simulink model "Modele_LQR_6DOF"  (R2025b)
settings: Solver=VariableStepAuto  StartTime=0.0  StopTime=300  FixedStep=0.033333  RelTol=1e-3
values from neighbouring files (symbols this model uses):
  B = -234.459    [AUV_Params.sldd]    (also in block_compute_K.m = [ [                                          0,             )
  Fx1 = -14.142    [AUV_Params.sldd]
  Fx2 = -14.142    [AUV_Params.sldd]
  Fx3 = 0.0    [AUV_Params.sldd]
  Fx4 = 0.0    [AUV_Params.sldd]
  Fx5 = 0.0    [AUV_Params.sldd]
  Fx6 = 0.0    [AUV_Params.sldd]
  Fx7 = 14.142    [AUV_Params.sldd]
  Fx8 = 14.142    [AUV_Params.sldd]
  Fy1 = 14.142    [AUV_Params.sldd]
  Fy2 = -14.142    [AUV_Params.sldd]
  Fy3 = 0.0    [AUV_Params.sldd]
  Fy4 = 0.0    [AUV_Params.sldd]
  Fy5 = 0.0    [AUV_Params.sldd]
  Fy6 = 0.0    [AUV_Params.sldd]
  Fy7 = 14.142    [AUV_Params.sldd]
  Fy8 = -14.142    [AUV_Params.sldd]
  Fz1 = 0.0    [AUV_Params.sldd]
  Fz2 = 0.0    [AUV_Params.sldd]
  Fz3 = -20.0    [AUV_Params.sldd]
  Fz4 = -20.0    [AUV_Params.sldd]
  Fz5 = -20.0    [AUV_Params.sldd]
  Fz6 = -20.0    [AUV_Params.sldd]
  Fz7 = 0.0    [AUV_Params.sldd]
  Fz8 = 0.0    [AUV_Params.sldd]
  I_x = 0.578    [AUV_Params.sldd]
  I_y = 0.645    [AUV_Params.sldd]
  I_z = 0.9366    [AUV_Params.sldd]
  lx1 = 0.0194    [AUV_Params.sldd]
  lx2 = 0.0194    [AUV_Params.sldd]
  lx3 = -0.0317    [AUV_Params.sldd]
  lx4 = -0.0317    [AUV_Params.sldd]
  lx5 = 0.0317    [AUV_Params.sldd]
  lx6 = 0.0317    [AUV_Params.sldd]
  lx7 = -0.0194    [AUV_Params.sldd]
  lx8 = -0.0194    [AUV_Params.sldd]
  ly1 = 0.0381    [AUV_Params.sldd]
  ly2 = -0.0381    [AUV_Params.sldd]
  ly3 = 0.0049    [AUV_Params.sldd]
  ly4 = -0.0049    [AUV_Params.sldd]
  ly5 = 0.0049    [AUV_Params.sldd]
  ly6 = -0.0049    [AUV_Params.sldd]
  ly7 = 0.0381    [AUV_Params.sldd]
  ly8 = -0.0381    [AUV_Params.sldd]
  lz1 = 0.0575    [AUV_Params.sldd]
  lz2 = 0.0575    [AUV_Params.sldd]
  lz3 = 0.0366    [AUV_Params.sldd]
  lz4 = 0.0366    [AUV_Params.sldd]
  lz5 = 0.0366    [AUV_Params.sldd]
  lz6 = 0.0366    [AUV_Params.sldd]
  lz7 = 0.0575    [AUV_Params.sldd]
  lz8 = 0.0575    [AUV_Params.sldd]
  m = 23.9    [AUV_Params.sldd]
  W = 234.459    [AUV_Params.sldd]
  x_rb = 0.0    [AUV_Params.sldd]
  x_rg = 0.0    [AUV_Params.sldd]
  y_rb = 0.0    [AUV_Params.sldd]
  y_rg = 0.0    [AUV_Params.sldd]
  z_rb = 0.0    [AUV_Params.sldd]
  z_rg = 0.0    [AUV_Params.sldd]
undefined symbols (not defined in the file or in its folder): A_num, Q_envoyer, sigbuilder_block, SIZE_TRAJ, T_TRAJ, TRAJECTOIRE, YAW_MODE
libraries: simulink x12, sharedtransform x1, dspinverses x1, SignalEditorBlockLib x1
(part 1 of 4)
settings Model: DataDictionary=AUV_Params.sldd  Creator=ASUQTR  LastModifiedBy=louis
settings SolverCC: ZeroCrossAlgorithm=Adaptive  AlgebraicLoopSolver=TrustRegion
settings DebuggingCC: IgnoredZcDiagnostic=none  UnconnectedInputMsg=warning  UnconnectedOutputMsg=warning  UnconnectedLineMsg=warning
settings ModelReferenceCC: EnableRefExpFcnMdlSchedulingChecks=on
settings RTWCC: GPUComputeCapability=3.5  DLArmComputeVersion=19.05

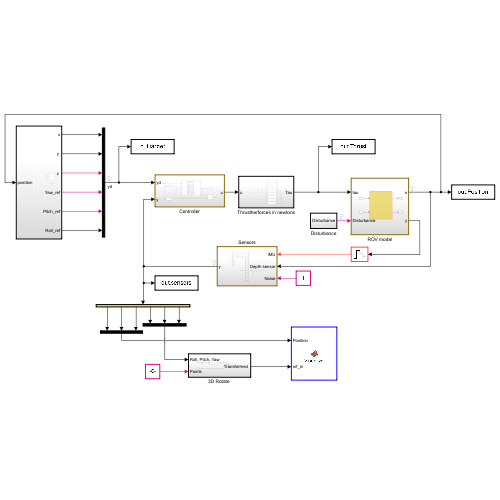
[thumbnail: Simulink's stored preview of the top-level diagram]
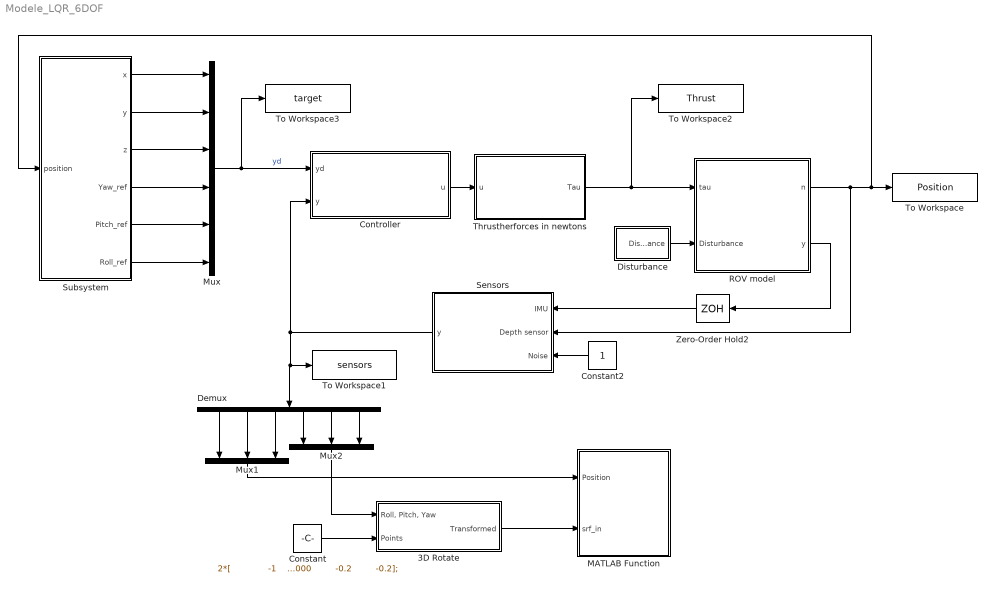
== system Modele_LQR_6DOF ==
  "3D Rotate " : Subsystem
  Constant : Constant  Value=|
      | 2*[              -1         -0.2         -0.2
      |     1.0000         -0.2         -0.2    
      | 1.0000    0.2000         -0.2
      |          -1    0.2000         -0.2
      |          -1         -0.2         -0.2
      |          -1         -0.2    0.2000
      |     1.0000         -0.2    0.2000
      |     1.0000    0.2000    0.2000
      |          -1    0.2000    0.2000
      |          -1         -0.2    0.2000
      |          -1   0.2000    0.2000
      |          -1    0.2000         -0.2
      |     1.0000    0.2000         -0.2
      |     1.0000    0.2000    0.2000
      |     1.0000         -0.2    0.2000
      |     1.0000         -0.2         -0.2];
  Constant2 : Constant
  Controller : Subsystem
  Demux : Demux  Outputs=6
  Disturbance : Subsystem
  MATLAB Function : MATLAB Function  TreatAsAtomicUnit=on  SystemSampleTime=0.05
  Mux : Mux  Inputs=6
  Mux1 : Mux  Inputs=3
  Mux2 : Mux  Inputs=3
  ROV model : Subsystem
  Sensors : Subsystem
  Subsystem : Subsystem
  Thrustherforces in newtons : Subsystem
  To Workspace : ToWorkspace  VariableName=Position  SaveFormat=Structure With Time  SampleTime=-1
  To Workspace1 : ToWorkspace  VariableName=sensors  SaveFormat=Structure With Time  SampleTime=-1
  To Workspace2 : ToWorkspace  VariableName=Thrust  SaveFormat=Structure With Time  SampleTime=-1
  To Workspace3 : ToWorkspace  VariableName=target  SaveFormat=Structure With Time  SampleTime=-1
  Zero-Order Hold2 : ZeroOrderHold  SampleTime=0.001
  wires:
  Mux/1 -> To Workspace3/1, Controller/1(yd)  "yd"
  Disturbance/1(Disturbance) -> ROV model/2(Disturbance)
  ROV model/1(n) -> Sensors/2(Depth sensor), Subsystem/1(position), To Workspace/1
  Thrustherforces in newtons/1(Tau) -> To Workspace2/1, ROV model/1(tau)
  Controller/1(u) -> Thrustherforces in newtons/1(u)
  Constant2/1 -> Sensors/3(Noise)
  Subsystem/2("y ") -> Mux/2
  Subsystem/1(x) -> Mux/1
  Subsystem/3("z ") -> Mux/3
  Subsystem/4(Yaw_ref) -> Mux/4
  Subsystem/5(Pitch_ref) -> Mux/5
  Subsystem/6(Roll_ref) -> Mux/6
  "3D Rotate "/1("Transformed ") -> MATLAB Function/2(srf_in)
  Constant/1 -> "3D Rotate "/2(Points)
  Demux/1 -> Mux1/1
  Demux/2 -> Mux1/2
  Demux/3 -> Mux1/3
  Mux1/1 -> MATLAB Function/1(Position)
  Demux/4 -> Mux2/1
  Demux/5 -> Mux2/2
  Demux/6 -> Mux2/3
  Mux2/1 -> "3D Rotate "/1("Roll, Pitch, Yaw")
  Sensors/1(y) -> To Workspace1/1, Demux/1, Controller/2(y)
  ROV model/2(y) -> Zero-Order Hold2/1
  Zero-Order Hold2/1 -> Sensors/1(IMU)

== system Modele_LQR_6DOF/3D Rotate  ==
  "Roll, Pitch, Yaw" : Inport
  Points : Inport  Port=2
  Gain : Gain
  Matrix Multiply : Product  Multiplication=Matrix(*)
  Rotation Angles to Direction Cosine Matrix : sharedtransform/Rotation Angles to Direction Cosine Matrix  rotationOrder=XYZ  aMode=aMode
  Transpose : Math  Operator=transpose  SignedPower=on
  "Transformed " : Outport  VectorParamsAs1DForOutWhenUnconnected=off
  wires:
  Matrix Multiply/1 -> "Transformed "/1
  Rotation Angles to Direction Cosine Matrix/1 -> Transpose/1
  Points/1 -> Matrix Multiply/1
  "Roll, Pitch, Yaw"/1 -> Gain/1
  Transpose/1 -> Matrix Multiply/2
  Gain/1 -> Rotation Angles to Direction Cosine Matrix/1

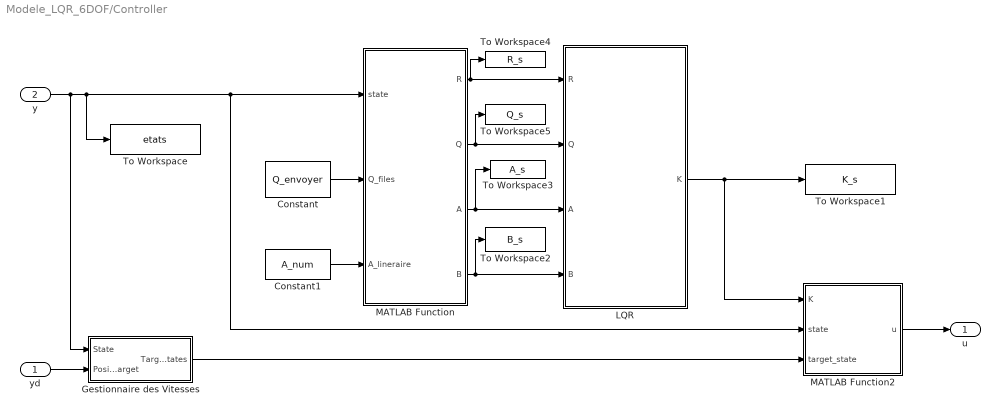
== system Modele_LQR_6DOF/Controller ==
  yd : Inport
  y : Inport  Port=2
  Constant : Constant  Value=Q_envoyer
  Constant1 : Constant  Value=A_num
  Gestionnaire des Vitesses : Subsystem
  LQR : Subsystem  Description=|  TreatAsAtomicUnit=on  mask(LQR with Algebric Riccati Equation){A=0, B=0, X0=0}
      | LQR Block
      | 
      | by Gurkan KAVURAN
      | gurkankavuran@gmail.com
      mask prompts: A "A (System Matrix)"; B "B (System Matrix)"; X0 "Xo (Initial Values of States)"
      mask help:
      | It is easy to optimize Q and R matrices with online process.
      | Please see the help file to define the block parameters.
      mask Help:
      | Parameters Example:
      | 
      | Q = diag([500 1 1 0 1 1] );
      | R = 1*diag([0.01 0.01 0.01 0.01]);
      | X0=[0 0 0 0 0 0;0 0 0 0 0 0;0 0 0 0 0 0;0 0 0 0 0 0;0 0 0 0 0 0;0 0 0 0 0 0];
      | 
      | "Matrix multiply" block is recommended to use in state feedback control mechanism.
      | 
      | 
      | http://www.gurkankavuran.com
      mask Display:
      | disp('LQR')
      | port_label('input', 1, 'R')
      | port_label('input', 2, 'Q')
      | port_label('input', 3, 'A')
      | port_label('input', 4, 'B')
      | port_label('output', 1, 'K')
  MATLAB Function : MATLAB Function  TreatAsAtomicUnit=on
  MATLAB Function2 : MATLAB Function  TreatAsAtomicUnit=on
  To Workspace : ToWorkspace  VariableName=etats  SaveFormat=Structure With Time  SampleTime=-1
  To Workspace1 : ToWorkspace  VariableName=K_s  SaveFormat=Structure With Time  SampleTime=-1
  To Workspace2 : ToWorkspace  VariableName=B_s  SaveFormat=Structure With Time  SampleTime=-1
  To Workspace3 : ToWorkspace  VariableName=A_s  SaveFormat=Structure With Time  SampleTime=-1
  To Workspace4 : ToWorkspace  VariableName=R_s  SaveFormat=Structure With Time  SampleTime=-1
  To Workspace5 : ToWorkspace  VariableName=Q_s  SaveFormat=Structure With Time  SampleTime=-1
  u : Outport
  wires:
  MATLAB Function/4(B) -> LQR/4(B), To Workspace2/1
  MATLAB Function/2(Q) -> LQR/2(Q), To Workspace5/1
  LQR/1(K) -> MATLAB Function2/1(K), To Workspace1/1
  y/1 -> Gestionnaire des Vitesses/1(State), To Workspace/1, MATLAB Function2/2(state), MATLAB Function/1(state)
  MATLAB Function/1(R) -> LQR/1(R), To Workspace4/1
  yd/1 -> Gestionnaire des Vitesses/2(Position_target)
  Gestionnaire des Vitesses/1(Target_states) -> MATLAB Function2/3(target_state)
  MATLAB Function/3(A) -> LQR/3(A), To Workspace3/1
  Constant/1 -> MATLAB Function/2(Q_files)
  Constant1/1 -> MATLAB Function/3(A_lineraire)
  MATLAB Function2/1(u) -> u/1

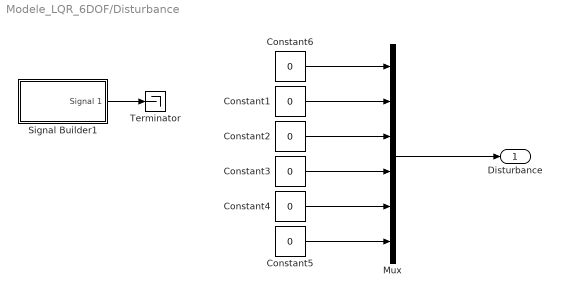
== system Modele_LQR_6DOF/Disturbance ==
  Constant{1..6} (6 alike) : Constant  Value=0
  Mux : Mux  Inputs=6
  Signal Builder1 : Subsystem  Tag=STV Subsys  LoadFcn=sigbuilder_block('load');  StartFcn=sigbuilder_block('start');  StopFcn=sigbuilder_block('stop');  ClipboardFcn=sigbuilder_block('clipboard');  mask(Sigbuilder block){tuvar=[0:10]}
      mask help: Simulink:masks:SigbuilderBlock_MD
      mask init:
      | if ~strcmp(get_param(bdroot(gcbh),'SimulationStatus'),'stopped') tuvar = sigbuilder_block('maskInit'); end
      settings: CopyFcn=sigbuilder_block('copy');  DeleteFcn=sigbuilder_block('delete');  ModelCloseFcn=sigbuilder_block('modelClose');  PreSaveFcn=sigbuilder_block('preSave');  PauseFcn=sigbuilder_block('pause');  ContinueFcn=sigbuilder_block('continue');  NameChangeFcn=sigbuilder_block('namechange');  OpenFcn=sigbuilder_block('open',[252.75 107.25 644.25 387.75 ]);  CloseFcn=sigbuilder_block('close');
      mask Display: plot(0, 0, 100, 100,[2, 2, 32, 32, 2], [68, 8, 8, 68, 68],[32, 2], [38, 38], [32, 19, 2],[53, 60, 44], [32, 17, 17, 2],[16, 16, 31, 31]);txt = getActiveGroup(gcbh);text(2, 100, txt,'verticalAlignment', 'top');
  Terminator : Terminator
  Disturbance : Outport
  wires:
  Mux/1 -> Disturbance/1
  Constant1/1 -> Mux/2
  Constant2/1 -> Mux/3
  Constant4/1 -> Mux/5
  Constant5/1 -> Mux/6
  Constant3/1 -> Mux/4
  Constant6/1 -> Mux/1
  Signal Builder1/1(Signal 1) -> Terminator/1

== system Modele_LQR_6DOF/ROV model ==
  tau : Inport
  Disturbance : Inport  Port=2
  ROV model : Subsystem
  n : Outport
  y : Outport  Port=2
  wires:
  tau/1 -> ROV model/1(tau)
  Disturbance/1 -> ROV model/2(Disturbance)
  ROV model/2(euler+vitesse_body) -> y/1
  ROV model/1(𝜂) -> n/1

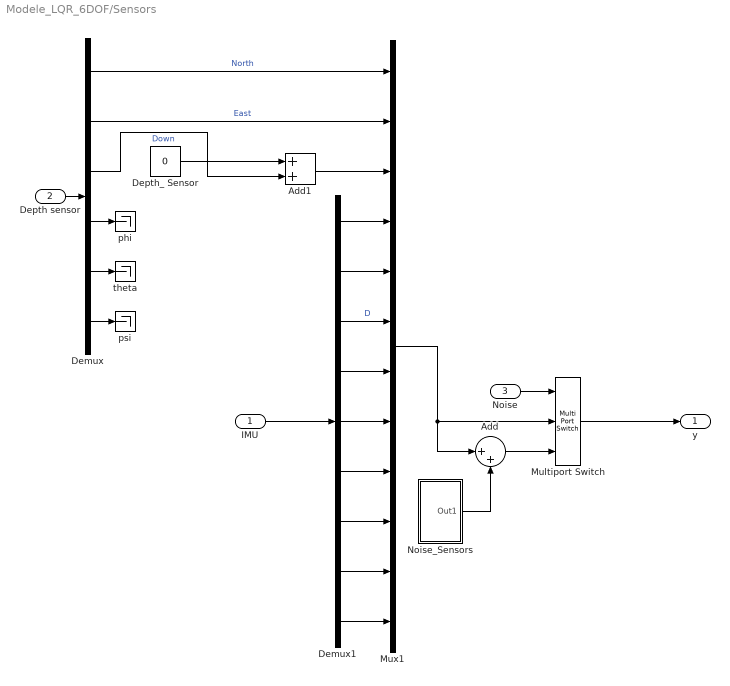
== system Modele_LQR_6DOF/Sensors ==
  IMU : Inport
  Depth sensor : Inport  Port=2
  Noise : Inport  Port=3
  Add : Sum  Inputs=|++
  Add1 : Sum
  Demux : Demux  Outputs=6
  Demux1 : Demux  Outputs=9
  Depth_ Sensor : Constant  Value=0
  Multiport Switch : MultiPortSwitch  Inputs=2  SaturateOnIntegerOverflow=off  InputSameDT=off
  Mux1 : Mux  Inputs=12
  Noise_Sensors : Subsystem
  phi : Terminator
  psi : Terminator
  theta : Terminator
  y : Outport
  wires:
  Multiport Switch/1 -> y/1
  Add/1 -> Multiport Switch/3
  Noise/1 -> Multiport Switch/1
  Mux1/1 -> Multiport Switch/2, Add/1
  Depth sensor/1 -> Demux/1
  Demux/4 -> phi/1
  Demux/5 -> theta/1
  Demux/6 -> psi/1
  Demux/3 -> Add1/2  "Down"
  Depth_ Sensor/1 -> Add1/1
  IMU/1 -> Demux1/1
  Add1/1 -> Mux1/3
  Demux/2 -> Mux1/2  "East"
  Demux/1 -> Mux1/1  "North"
  Demux1/1 -> Mux1/4
  Demux1/2 -> Mux1/5
  Demux1/3 -> Mux1/6  "D"
  Demux1/4 -> Mux1/7
  Demux1/5 -> Mux1/8
  Demux1/6 -> Mux1/9
  Demux1/7 -> Mux1/10
  Demux1/8 -> Mux1/11
  Demux1/9 -> Mux1/12
  Noise_Sensors/1(Out1) -> Add/2

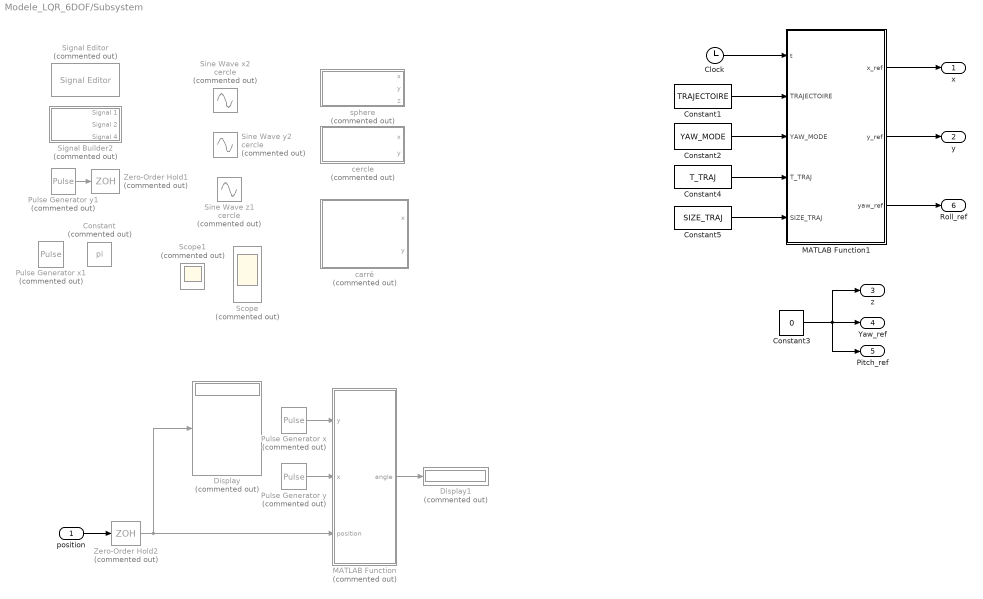
== system Modele_LQR_6DOF/Subsystem ==
  position : Inport
  Clock : Clock
  Constant : Constant  Commented=on  Value=pi
  Constant1 : Constant  Value=TRAJECTOIRE
  Constant2 : Constant  Value=YAW_MODE
  Constant3 : Constant  Value=0
  Constant4 : Constant  Value=T_TRAJ
  Constant5 : Constant  Value=SIZE_TRAJ
  Display : Display  Commented=on
  Display1 : Display  Commented=on
  MATLAB Function : MATLAB Function  Commented=on  TreatAsAtomicUnit=on
  MATLAB Function1 : MATLAB Function  TreatAsAtomicUnit=on
  Pulse Generator x : DiscretePulseGenerator  Commented=on  PulseType=Time based  Amplitude=2  Period=30  PulseWidth=50
  Pulse Generator x1 : DiscretePulseGenerator  Commented=on  PulseType=Time based  Amplitude=pi  Period=30  PulseWidth=50
  Pulse Generator y : DiscretePulseGenerator  Commented=on  PulseType=Time based  Amplitude=2  Period=30  PulseWidth=50  PhaseDelay=7.5
  Pulse Generator y1 : DiscretePulseGenerator  Commented=on  PulseType=Time based  Amplitude=pi/2  Period=30  PulseWidth=50  PhaseDelay=7.5
  Scope : Scope  Commented=on  NumInputPorts=3
      settings: ActiveDisplayYMinimum=-0.25  ActiveDisplayYMaximum=2.25
  Scope1 : Scope  Commented=on  NumInputPorts=2
      settings: ActiveDisplayYMinimum=-1  ActiveDisplayYMaximum=1
  Signal Builder2 : Subsystem  Tag=STV Subsys  Commented=on  LoadFcn=sigbuilder_block('load');  StartFcn=sigbuilder_block('start');  StopFcn=sigbuilder_block('stop');  ClipboardFcn=sigbuilder_block('clipboard');  mask(Sigbuilder block){tuvar=[0:10]}
      mask help: Simulink:masks:SigbuilderBlock_MD
      mask init:
      | if ~strcmp(get_param(bdroot(gcbh),'SimulationStatus'),'stopped') tuvar = sigbuilder_block('maskInit'); end
      settings: CopyFcn=sigbuilder_block('copy');  DeleteFcn=sigbuilder_block('delete');  ModelCloseFcn=sigbuilder_block('modelClose');  PreSaveFcn=sigbuilder_block('preSave');  PauseFcn=sigbuilder_block('pause');  ContinueFcn=sigbuilder_block('continue');  NameChangeFcn=sigbuilder_block('namechange');  OpenFcn=sigbuilder_block('open',[566.25 108.75 550.5 372.75 ]);  CloseFcn=sigbuilder_block('close');
      mask Display: plot(0, 0, 100, 100,[2, 2, 32, 32, 2], [68, 8, 8, 68, 68],[32, 2], [38, 38], [32, 19, 2],[53, 60, 44], [32, 17, 17, 2],[16, 16, 31, 31]);txt = getActiveGroup(gcbh);text(2, 100, txt,'verticalAlignment', 'top');
  Signal Editor : SignalEditorBlockLib/Signal Editor  Commented=on  FileName=sous marin en pentagone.mat  ActiveScenario=Scenario  ActiveSignal=Signal X  IsBus=off  OutputBusObjectStr=Bus: BusObject  SampleTime=0  Interpolate=off  ZeroCross=off  OutputAfterFinalValue=Setting to zero  Unit=inherit  PreserveSignalName=on  ApplySigPropsToAllScenarios=on  ApplySigPropsToAllSignals=off  SignalPropertySource=Dialog parameters
  Sine Wave x2 cercle : Sin  Commented=on  Amplitude=2  Frequency=0.48541  Phase=pi/2  SampleTime=0
  Sine Wave y2 cercle : Sin  Commented=on  Amplitude=2  Frequency=0.48541  SampleTime=0
  Sine Wave z1 cercle : Sin  Commented=on  Amplitude=2  Frequency=0.3  Phase=pi/2  SampleTime=0
  Zero-Order Hold1 : ZeroOrderHold  Commented=on  SampleTime=8
  Zero-Order Hold2 : ZeroOrderHold  Commented=on
  carré : Subsystem  Commented=on
  cercle : Subsystem  Commented=on
  sphere : Subsystem  Commented=on
  x : Outport  VectorParamsAs1DForOutWhenUnconnected=off
  "y " : Outport  Port=2  VectorParamsAs1DForOutWhenUnconnected=off
  "z " : Outport  Port=3  VectorParamsAs1DForOutWhenUnconnected=off
  Yaw_ref : Outport  Port=4  VectorParamsAs1DForOutWhenUnconnected=off
  Pitch_ref : Outport  Port=5  VectorParamsAs1DForOutWhenUnconnected=off
  Roll_ref : Outport  Port=6  VectorParamsAs1DForOutWhenUnconnected=off
  wires:
  Pulse Generator x/1 -> MATLAB Function/1(y)
  position/1 -> Zero-Order Hold2/1
  Zero-Order Hold2/1 -> Display/1, MATLAB Function/3(position)
  MATLAB Function/1(angle) -> Display1/1
  Pulse Generator y/1 -> MATLAB Function/2(x)
  Pulse Generator y1/1 -> Zero-Order Hold1/1
  Constant3/1 -> Yaw_ref/1, "z "/1, Pitch_ref/1
  Clock/1 -> MATLAB Function1/1(t)
  MATLAB Function1/1(x_ref) -> x/1
  MATLAB Function1/2(y_ref) -> "y "/1
  Constant1/1 -> MATLAB Function1/2(TRAJECTOIRE)
  Constant2/1 -> MATLAB Function1/3(YAW_MODE)
  MATLAB Function1/3(yaw_ref) -> Roll_ref/1
  Constant4/1 -> MATLAB Function1/4(T_TRAJ)
  Constant5/1 -> MATLAB Function1/5(SIZE_TRAJ)

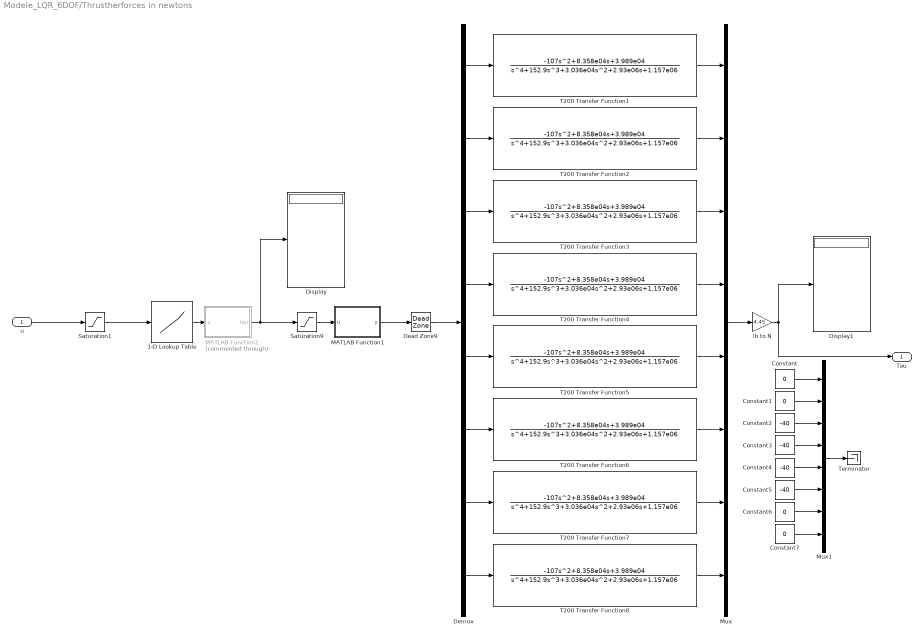
== system Modele_LQR_6DOF/Thrustherforces in newtons ==
  u : Inport
  1-D Lookup Table : Lookup_n-D  NumberOfTableDimensions=1  BreakpointsForDimension1=[-1:0.01:1]  Table=1500 + 400 * ([-1:0.01:1])  InternalRulePriority=Speed  RndMeth=Simplest
  Constant{,1,6..7} (4 alike) : Constant  Value=0
  Constant{2..5} (4 alike) : Constant  Value=-40
  Dead Zone9 : DeadZone  LowerValue=-10  UpperValue=+10
  Demux : Demux  Outputs=8
  Display : Display
  Display1 : Display
  MATLAB Function1 : MATLAB Function  TreatAsAtomicUnit=on
  MATLAB Function2 : MATLAB Function  Commented=through  TreatAsAtomicUnit=on
  Mux : Mux  Inputs=8
  Mux1 : Mux  Inputs=8
  Saturation1 : Saturate  UpperLimit=1  LowerLimit=-1
  Saturation9 : Saturate  UpperLimit=1900  LowerLimit=1100
  T200 Transfer Function{1..8} (8 alike) : TransferFcn  Numerator="[-107  8.358e04  3.989e04]"  Denominator="[1 152.9  3.036e04  2.93e06  1.157e06]"
  Terminator : Terminator
  lb to N : Gain  Gain=4.45
  Tau : Outport
  wires:
  u/1 -> Saturation1/1
  1-D Lookup Table/1 -> MATLAB Function2/1(u)
  Dead Zone9/1 -> Demux/1
  T200 Transfer Function1/1 -> Mux/1
  T200 Transfer Function5/1 -> Mux/5
  T200 Transfer Function7/1 -> Mux/7
  T200 Transfer Function8/1 -> Mux/8
  Mux/1 -> lb to N/1
  lb to N/1 -> Display1/1, Tau/1
  Saturation9/1 -> MATLAB Function1/1(u)
  MATLAB Function1/1(y) -> Dead Zone9/1
  MATLAB Function2/1(tau) -> Display/1, Saturation9/1
  Constant/1 -> Mux1/1
  Constant1/1 -> Mux1/2
  Constant2/1 -> Mux1/3
  Constant3/1 -> Mux1/4
  Constant4/1 -> Mux1/5
  Constant5/1 -> Mux1/6
  Constant6/1 -> Mux1/7
  Constant7/1 -> Mux1/8
  Demux/1 -> T200 Transfer Function1/1
  Demux/2 -> T200 Transfer Function2/1
  Demux/3 -> T200 Transfer Function3/1
  Demux/4 -> T200 Transfer Function4/1
  Demux/5 -> T200 Transfer Function5/1
  Demux/6 -> T200 Transfer Function6/1
  Demux/7 -> T200 Transfer Function7/1
  Demux/8 -> T200 Transfer Function8/1
  T200 Transfer Function6/1 -> Mux/6
  T200 Transfer Function2/1 -> Mux/2
  T200 Transfer Function3/1 -> Mux/3
  T200 Transfer Function4/1 -> Mux/4
  Saturation1/1 -> 1-D Lookup Table/1
  Mux1/1 -> Terminator/1

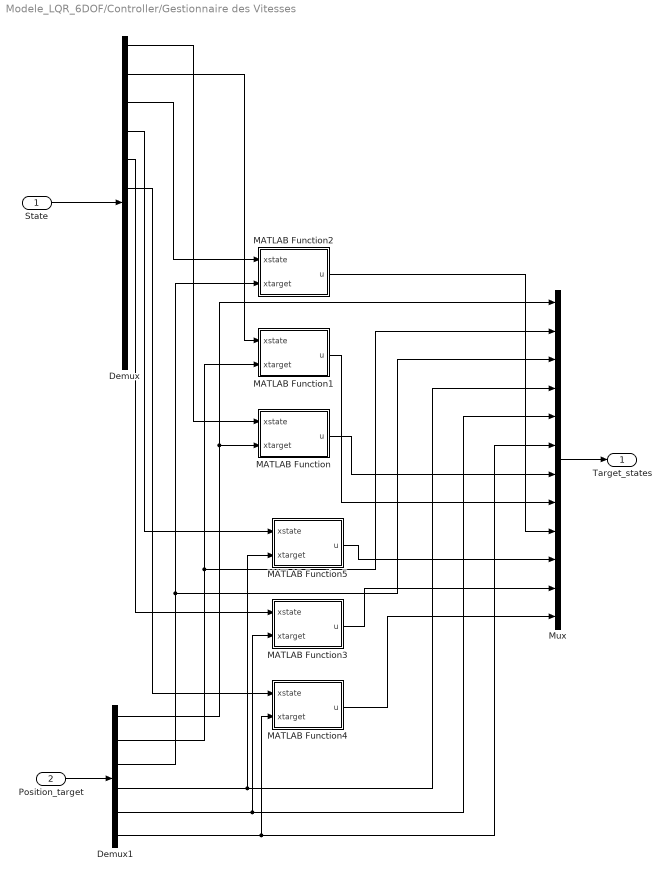
== system Modele_LQR_6DOF/Controller/Gestionnaire des Vitesses ==
  State : Inport
  Position_target : Inport  Port=2
  Demux : Demux  Outputs=12
  Demux1 : Demux  Outputs=6
  MATLAB Function : MATLAB Function  TreatAsAtomicUnit=on
  MATLAB Function1 : MATLAB Function  TreatAsAtomicUnit=on
  MATLAB Function2 : MATLAB Function  TreatAsAtomicUnit=on
  MATLAB Function3 : MATLAB Function  TreatAsAtomicUnit=on
  MATLAB Function4 : MATLAB Function  TreatAsAtomicUnit=on
  MATLAB Function5 : MATLAB Function  TreatAsAtomicUnit=on
  Mux : Mux  Inputs=12
  Target_states : Outport
  wires:
  State/1 -> Demux/1
  Position_target/1 -> Demux1/1
  Mux/1 -> Target_states/1
  Demux1/4 -> MATLAB Function5/2(xtarget), Mux/4
  Demux1/5 -> MATLAB Function3/2(xtarget), Mux/5
  Demux1/6 -> MATLAB Function4/2(xtarget), Mux/6
  Demux1/2 -> MATLAB Function1/2(xtarget), Mux/2
  Demux1/3 -> MATLAB Function2/2(xtarget), Mux/3
  MATLAB Function2/1(u) -> Mux/9
  MATLAB Function1/1(u) -> Mux/8
  Demux/1 -> MATLAB Function/1(xstate)
  Demux1/1 -> Mux/1, MATLAB Function/2(xtarget)
  MATLAB Function/1(u) -> Mux/7
  Demux/2 -> MATLAB Function1/1(xstate)
  Demux/3 -> MATLAB Function2/1(xstate)
  Demux/4 -> MATLAB Function5/1(xstate)
  Demux/5 -> MATLAB Function3/1(xstate)
  Demux/6 -> MATLAB Function4/1(xstate)
  MATLAB Function4/1(u) -> Mux/12
  MATLAB Function3/1(u) -> Mux/11
  MATLAB Function5/1(u) -> Mux/10

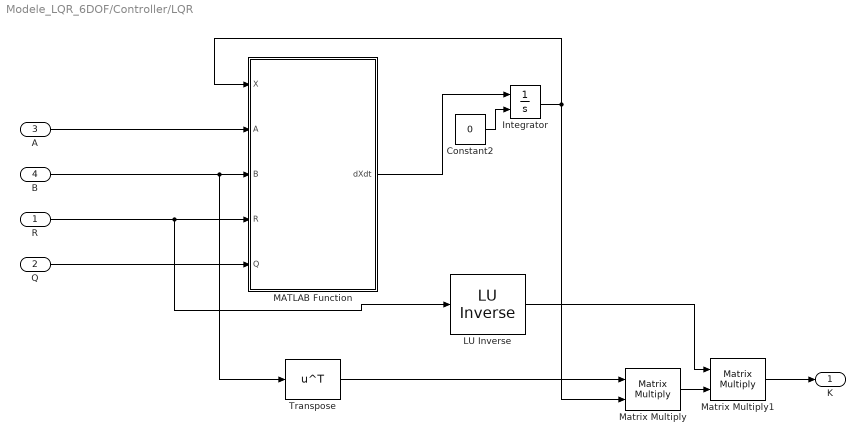
== system Modele_LQR_6DOF/Controller/LQR ==
  R : Inport
  Q : Inport  Port=2
  A : Inport  Port=3
  B : Inport  Port=4
  " LU Inverse" : dspinverses/ LU Inverse
  Constant2 : Constant  Value=0
  Integrator : Integrator  InitialConditionSource=external  InitialCondition=[1 1 1 1 1 1 1 1 1 1 1 1 1 1 1 1 1 1 1 1 1 1 1 1 1 1 1 1 1 1 1 1 1 1 1 1]
  MATLAB Function : MATLAB Function  TreatAsAtomicUnit=on
  Matrix Multiply : Product  Multiplication=Matrix(*)
  Matrix Multiply1 : Product  Multiplication=Matrix(*)
  Transpose : Math  Operator=transpose
  K : Outport
  wires:
  Matrix Multiply1/1 -> K/1
  A/1 -> MATLAB Function/2(A)
  B/1 -> Transpose/1, MATLAB Function/3(B)
  " LU Inverse"/1 -> Matrix Multiply1/1
  Constant2/1 -> Integrator/2
  Matrix Multiply/1 -> Matrix Multiply1/2
  Transpose/1 -> Matrix Multiply/1
  Integrator/1 -> Matrix Multiply/2, MATLAB Function/1(X)
  Q/1 -> MATLAB Function/5(Q)
  R/1 -> " LU Inverse"/1, MATLAB Function/4(R)
  MATLAB Function/1(dXdt) -> Integrator/1

== system Modele_LQR_6DOF/Disturbance/Signal Builder1 ==
  Demux : Demux  Tag=STV Demux  Outputs=1
      settings: DisplayOption=none
  FromWs : FromWorkspace  Tag=STV FromWs  VariableName=tuvar
      SigBuilderData=|
      | common.afterFinalStr = 'Extrapolate'
      | common.sampleTime = 0
      | dataSet.timeRange = [0 20]
      | dataSet.name = 'Group 1'
      | sbobj.Groups.Name = 'Group 1'
      | sbobj.Groups.Signals.Name = 'Signal 1'
      | sbobj.Groups.Signals.XData = [0 2 20]
      | sbobj.Groups.Signals.YData = [0 1 1]
      | sbobj.Groups.TimeRange = [0 20]
  Signal 1 : Outport  Tag=STV Outport
  wires:
  FromWs/1 -> Demux/1
  Demux/1 -> Signal 1/1

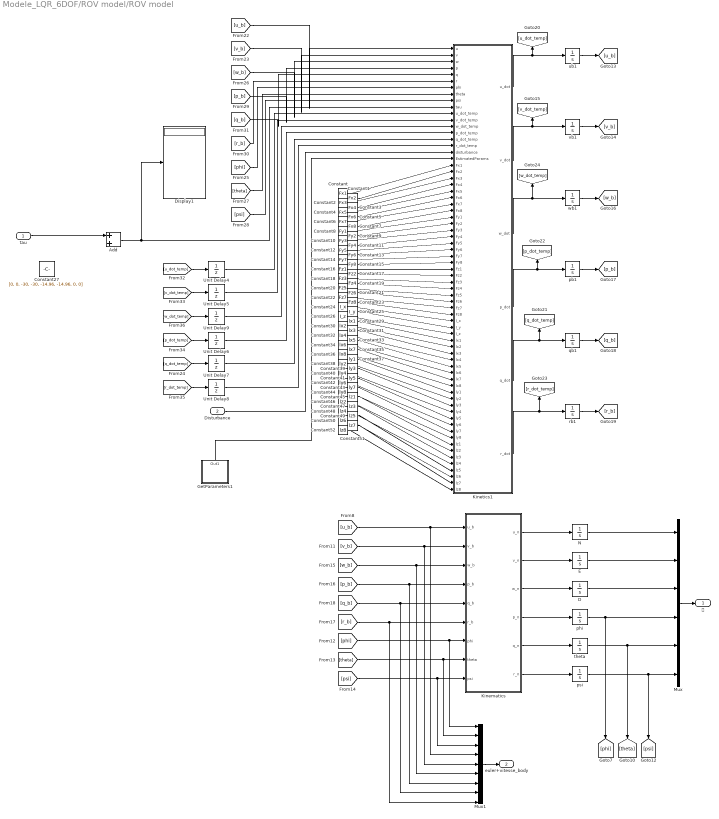
== system Modele_LQR_6DOF/ROV model/ROV model ==
  tau : Inport
  Disturbance : Inport  Port=2
  Add : Sum
  Constant : Constant  Value=Fx1
  Constant1 : Constant  Value=Fx2
  Constant10 : Constant  Value=Fy3
  Constant11 : Constant  Value=Fy4
  Constant12 : Constant  Value=Fy5
  Constant13 : Constant  Value=Fy6
  Constant14 : Constant  Value=Fy7
  Constant15 : Constant  Value=Fy8
  Constant16 : Constant  Value=Fz1
  Constant17 : Constant  Value=Fz2
  Constant18 : Constant  Value=Fz3
  Constant19 : Constant  Value=Fz4
  Constant2 : Constant  Value=Fx3
  Constant20 : Constant  Value=Fz5
  Constant21 : Constant  Value=Fz6
  Constant22 : Constant  Value=Fz7
  Constant23 : Constant  Value=Fz8
  Constant24 : Constant  Value=I_x
  Constant25 : Constant  Value=I_y
  Constant26 : Constant  Value=I_z
  Constant27 : Constant  Value=[0, 0, -30, -30, -14.96, -14.96, 0, 0]
  Constant29 : Constant  Value=lx1
  Constant3 : Constant  Value=Fx4
  Constant30 : Constant  Value=lx2
  Constant31 : Constant  Value=lx3
  Constant32 : Constant  Value=lx4
  Constant33 : Constant  Value=lx5
  Constant34 : Constant  Value=lx6
  Constant35 : Constant  Value=lx7
  Constant36 : Constant  Value=lx8
  Constant37 : Constant  Value=ly1
  Constant38 : Constant  Value=ly2
  Constant39 : Constant  Value=ly3
  Constant4 : Constant  Value=Fx5
  Constant40 : Constant  Value=ly4
  Constant41 : Constant  Value=ly5
  Constant42 : Constant  Value=ly6
  Constant43 : Constant  Value=ly7
  Constant44 : Constant  Value=ly8
  Constant45 : Constant  Value=lz1
  Constant46 : Constant  Value=lz2
  Constant47 : Constant  Value=lz3
  Constant48 : Constant  Value=lz4
  Constant49 : Constant  Value=lz5
  Constant5 : Constant  Value=Fx6
  Constant50 : Constant  Value=lz6
  Constant51 : Constant  Value=lz7
  Constant52 : Constant  Value=lz8
  Constant6 : Constant  Value=Fx7
  Constant7 : Constant  Value=Fx8
  Constant8 : Constant  Value=Fy1
  Constant9 : Constant  Value=Fy2
  D : Integrator  InitialCondition=0.0000001  ContinuousStateAttributes='phi'
  Display1 : Display
  E : Integrator  InitialCondition=0.0000001  ContinuousStateAttributes='phi'
  GetParameters1 : Subsystem
  Kinematics : MATLAB Function  TreatAsAtomicUnit=on
  Kinetics1 : MATLAB Function  TreatAsAtomicUnit=on
  Mux : Mux  Inputs=6
  Mux1 : Mux  Inputs=9
  N : Integrator  InitialCondition=0.0000001  ContinuousStateAttributes='phi'
  Unit Delay{4..9} (6 alike) : UnitDelay  SampleTime=0.01  HasFrameUpgradeWarning=on
  pb1 : Integrator  InitialCondition=0.0000001
  phi : Integrator  InitialCondition=0.0000001  ContinuousStateAttributes='phi'
  psi : Integrator  InitialCondition=0.0000001  ContinuousStateAttributes='psi'
  qb1 : Integrator  InitialCondition=0.0000001
  rb1 : Integrator  InitialCondition=0.0000001
  theta : Integrator  InitialCondition=0.0000001  ContinuousStateAttributes='theta'
  ub1 : Integrator  InitialCondition=0.0000001
  vb1 : Integrator  InitialCondition=0.0000001
  wb1 : Integrator  InitialCondition=0.0000001
  𝜂 : Outport
  euler+vitesse_body : Outport  Port=2
  wires:
  Unit Delay9/1 -> Kinetics1/13(w_dot_temp)
  [phi] -> Kinetics1/7(phi)
  Kinetics1/4(p_dot) -> [p_dot_temp], pb1/1
  [w_dot_temp] -> Unit Delay9/1
  Kinetics1/2(v_dot) -> [v_dot_temp], vb1/1
  [r_b] -> Kinetics1/6(r)
  Kinetics1/6(r_dot) -> rb1/1, [r_dot_temp]
  Unit Delay8/1 -> Kinetics1/16(r_dot_temp)
  [u_b] -> Kinetics1/1(u)
  Unit Delay7/1 -> Kinetics1/15(q_dot_temp)
  rb1/1 -> [r_b]
  Unit Delay6/1 -> Kinetics1/14(p_dot_temp)
  [q_b] -> Kinetics1/5(q)
  [r_dot_temp] -> Unit Delay8/1
  [psi] -> Kinetics1/9(psi)
  [p_dot_temp] -> Unit Delay6/1
  [q_dot_temp] -> Unit Delay7/1
  [p_b] -> Kinetics1/4(p)
  Disturbance/1 -> Kinetics1/17(disturbance)
  Kinetics1/1(u_dot) -> [u_dot_temp], ub1/1
  Unit Delay5/1 -> Kinetics1/12(v_dot_temp)
  [theta] -> Kinetics1/8(theta)
  Kinetics1/5(q_dot) -> qb1/1, [q_dot_temp]
  [v_b] -> Kinetics1/2(v)
  GetParameters1/1(Out1) -> Kinetics1/18(EstimatedParams)
  [w_b] -> Kinetics1/3(w)
  pb1/1 -> [p_b]
  [v_dot_temp] -> Unit Delay5/1
  qb1/1 -> [q_b]
  vb1/1 -> [v_b]
  ub1/1 -> [u_b]
  wb1/1 -> [w_b]
  Kinetics1/3(w_dot) -> [w_dot_temp], wb1/1
  [u_dot_temp] -> Unit Delay4/1
  Unit Delay4/1 -> Kinetics1/11(u_dot_temp)
  [r_b] -> Mux1/9, Kinematics/6(r_b)
  [w_b] -> Mux1/6, Kinematics/3(w_b)
  Kinematics/4(p_n) -> phi/1
  Mux1/1 -> euler+vitesse_body/1
  phi/1 -> Mux/4, [phi]
  Kinematics/5(q_n) -> theta/1
  psi/1 -> Mux/6, [psi]
  [phi] -> Mux1/1, Kinematics/7(phi)
  Kinematics/1(u_n) -> N/1
  [theta] -> Mux1/2, Kinematics/8(theta)
  Kinematics/6(r_n) -> psi/1
  Kinematics/3(w_n) -> D/1
  D/1 -> Mux/3
  E/1 -> Mux/2
  [q_b] -> Mux1/8, Kinematics/5(q_b)
  [u_b] -> Mux1/4, Kinematics/1(u_b)
  [v_b] -> Mux1/5, Kinematics/2(v_b)
  theta/1 -> Mux/5, [theta]
  [p_b] -> Mux1/7, Kinematics/4(p_b)
  [psi] -> Mux1/3, Kinematics/9(psi)
  Kinematics/2(v_n) -> E/1
  Mux/1 -> 𝜂/1
  Constant/1 -> Kinetics1/19(Fx1)
  Constant1/1 -> Kinetics1/20(Fx2)
  Constant2/1 -> Kinetics1/21(Fx3)
  Constant3/1 -> Kinetics1/22(Fx4)
  Constant4/1 -> Kinetics1/23(Fx5)
  Constant5/1 -> Kinetics1/24(Fx6)
  Constant6/1 -> Kinetics1/25(Fx7)
  Constant7/1 -> Kinetics1/26(Fx8)
  Constant8/1 -> Kinetics1/27(Fy1)
  Constant9/1 -> Kinetics1/28(Fy2)
  Constant10/1 -> Kinetics1/29(Fy3)
  Constant11/1 -> Kinetics1/30(Fy4)
  Constant12/1 -> Kinetics1/31(Fy5)
  Constant13/1 -> Kinetics1/32(Fy6)
  Constant14/1 -> Kinetics1/33(Fy7)
  Constant15/1 -> Kinetics1/34(Fy8)
  Constant16/1 -> Kinetics1/35(Fz1)
  Constant17/1 -> Kinetics1/36(Fz2)
  Constant18/1 -> Kinetics1/37(Fz3)
  Constant19/1 -> Kinetics1/38(Fz4)
  Constant20/1 -> Kinetics1/39(Fz5)
  Constant21/1 -> Kinetics1/40(Fz6)
  Constant22/1 -> Kinetics1/41(Fz7)
  Constant23/1 -> Kinetics1/42(Fz8)
  Constant24/1 -> Kinetics1/43(I_x)
  Constant25/1 -> Kinetics1/44(I_y)
  Constant26/1 -> Kinetics1/45(I_z)
  Constant34/1 -> Kinetics1/51(lx6)
  Constant33/1 -> Kinetics1/50(lx5)
  Constant35/1 -> Kinetics1/52(lx7)
  Constant31/1 -> Kinetics1/48(lx3)
  Constant32/1 -> Kinetics1/49(lx4)
  Constant30/1 -> Kinetics1/47(lx2)
  Constant29/1 -> Kinetics1/46(lx1)
  Constant36/1 -> Kinetics1/53(lx8)
  Constant38/1 -> Kinetics1/55(ly2)
  Constant37/1 -> Kinetics1/54(ly1)
  Constant44/1 -> Kinetics1/61(ly8)
  Constant43/1 -> Kinetics1/60(ly7)
  Constant45/1 -> Kinetics1/62(lz1)
  Constant41/1 -> Kinetics1/58(ly5)
  Constant42/1 -> Kinetics1/59(ly6)
  Constant40/1 -> Kinetics1/57(ly4)
  Constant39/1 -> Kinetics1/56(ly3)
  Constant46/1 -> Kinetics1/63(lz2)
  Constant48/1 -> Kinetics1/65(lz4)
  Constant47/1 -> Kinetics1/64(lz3)
  Constant51/1 -> Kinetics1/68(lz7)
  Constant52/1 -> Kinetics1/69(lz8)
  Constant50/1 -> Kinetics1/67(lz6)
  Constant49/1 -> Kinetics1/66(lz5)
  N/1 -> Mux/1
  tau/1 -> Add/1
  Add/1 -> Kinetics1/10(tau), Display1/1

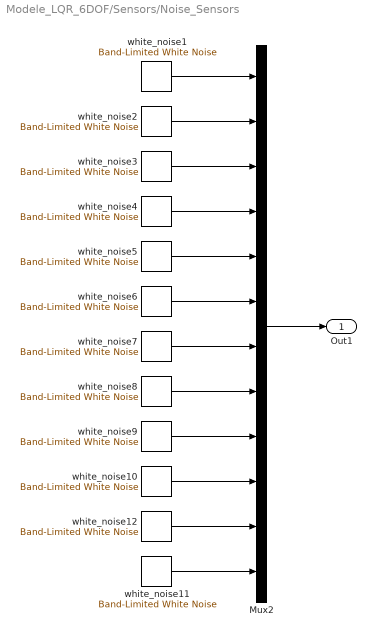
== system Modele_LQR_6DOF/Sensors/Noise_Sensors ==
  Mux2 : Mux  Inputs=12
  white_noise1 : simulink/Sources/Band-Limited White Noise  Cov=0.000010  Ts=0.01  seed=[23341]
  white_noise{7..12} (6 alike) : simulink/Sources/Band-Limited White Noise  Cov=0.000010  Ts=0.010000  seed=[8093341]
  white_noise2 : simulink/Sources/Band-Limited White Noise  Cov=0.000010  Ts=0.010000  seed=[23312341]
  white_noise3 : simulink/Sources/Band-Limited White Noise  Cov=0.000010  Ts=0.010000  seed=[2334571]
  white_noise4 : simulink/Sources/Band-Limited White Noise  Cov=0.000010  Ts=0.010000  seed=[21344441]
  white_noise5 : simulink/Sources/Band-Limited White Noise  Cov=0.000010  Ts=0.010000  seed=[3304141]
  white_noise6 : simulink/Sources/Band-Limited White Noise  Cov=0.000010  Ts=0.010000  seed=[903341]
  Out1 : Outport
  wires:
  white_noise10/1 -> Mux2/10
  white_noise8/1 -> Mux2/8
  white_noise7/1 -> Mux2/7
  white_noise11/1 -> Mux2/12
  white_noise2/1 -> Mux2/2
  white_noise12/1 -> Mux2/11
  white_noise5/1 -> Mux2/5
  white_noise1/1 -> Mux2/1
  white_noise3/1 -> Mux2/3
  white_noise6/1 -> Mux2/6
  white_noise9/1 -> Mux2/9
  white_noise4/1 -> Mux2/4
  Mux2/1 -> Out1/1

== system Modele_LQR_6DOF/Subsystem/Signal Builder2 ==
  Demux : Demux  Tag=STV Demux  Outputs=3
      settings: DisplayOption=none
  FromWs : FromWorkspace  Tag=STV FromWs  VariableName=tuvar
      SigBuilderData=|
      | common.afterFinalStr = 'Extrapolate'
      | common.sampleTime = 0
      | dataSet(1).timeRange = [0 50]
      | dataSet(1).name = 'Group 2'
      | dataSet(2).timeRange = [0 50]
      | dataSet(2).name = 'Group 1'
      | sbobj.Groups(1).Name = 'Group 2'
      | sbobj.Groups(1).Signals(1).Name = 'Signal 1'
      | sbobj.Groups(1).Signals(1).XData = [0 2 25 26 50]
      | sbobj.Groups(1).Signals(1).YData = [0 2 2 0 0]
      | sbobj.Groups(1).Signals(2).Name = 'Signal 2'
      | sbobj.Groups(1).Signals(2).XData = [0 12 13 37 38 50]
      | sbobj.Groups(1).Signals(2).YData = [0 0 2 2 0 0]
      | sbobj.Groups(1).Signals(3).Name = 'Signal 4'
      | sbobj.Groups(1).Signals(3).XData = [0 20 20 30 30 50]
      | sbobj.Groups(1).Signals(3).YData = [0 0 1 1 0 0]
      | sbobj.Groups(1).TimeRange = [0 50]
      | sbobj.Groups(2).Name = 'Group 1'
      | sbobj.Groups(2).Signals(1).Name = 'Signal 1'
      | sbobj.Groups(2).Signals(1).XData = [0 2 25 26 50]
      | sbobj.Groups(2).Signals(1).YData = [0 2 2 0 0]
      | sbobj.Groups(2).Signals(2).Name = 'Signal 2'
      | sbobj.Groups(2).Signals(2).XData = [0 12 13 37 38 50]
      | sbobj.Groups(2).Signals(2).YData = [0 0 2 2 0 0]
      | sbobj.Groups(2).Signals(3).Name = 'Signal 4'
      | sbobj.Groups(2).Signals(3).XData = [0 5.2 5.2 30 50]
      | sbobj.Groups(2).Signals(3).YData = [0 0.98 1 1 0.01]
      | sbobj.Groups(2).TimeRange = [0 50]
  Signal 1 : Outport  Tag=STV Outport
  Signal 2 : Outport  Tag=STV Outport  Port=2
  Signal 4 : Outport  Tag=STV Outport  Port=3
  wires:
  FromWs/1 -> Demux/1
  Demux/1 -> Signal 1/1
  Demux/2 -> Signal 2/1
  Demux/3 -> Signal 4/1

== system Modele_LQR_6DOF/Subsystem/carré ==
  Pulse Generator x : DiscretePulseGenerator  PulseType=Time based  Amplitude=2  Period=30  PulseWidth=50  PhaseDelay=1.5
  Pulse Generator y : DiscretePulseGenerator  PulseType=Time based  Amplitude=2  Period=30  PulseWidth=50  PhaseDelay=8.5
  x : Outport
  y : Outport  Port=2
  wires:
  Pulse Generator x/1 -> x/1
  Pulse Generator y/1 -> y/1

== system Modele_LQR_6DOF/Subsystem/cercle ==
  note: pour temps de 50s
      | rad/s = 0.12566
  Constant : Constant  Value=2
  Sine Wave x1 cercle : Sin  Amplitude=2  Frequency=0.12566  SampleTime=0
  Sine Wave y1 cercle : Sin  Amplitude=2  Frequency=0.12566  Phase=pi/2  SampleTime=0
  Subtract : Sum  Inputs=+-
  x : Outport
  y : Outport  Port=2
  wires:
  Sine Wave y1 cercle/1 -> Subtract/1
  Constant/1 -> Subtract/2
  Subtract/1 -> y/1
  Sine Wave x1 cercle/1 -> x/1

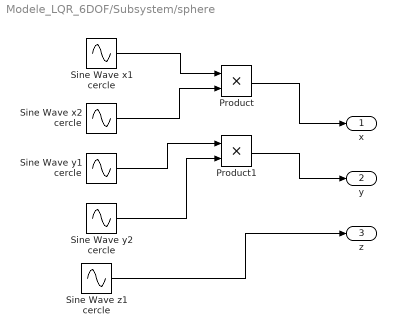
== system Modele_LQR_6DOF/Subsystem/sphere ==
  Product : Product
  Product1 : Product
  Sine Wave x1 cercle : Sin  Amplitude=2  Frequency=0.3  SampleTime=0
  Sine Wave x2 cercle : Sin  Amplitude=2  Frequency=0.48541  Phase=pi/2  SampleTime=0
  Sine Wave y1 cercle : Sin  Amplitude=2  Frequency=0.3  SampleTime=0
  Sine Wave y2 cercle : Sin  Amplitude=2  Frequency=0.48541  SampleTime=0
  Sine Wave z1 cercle : Sin  Amplitude=2  Frequency=0.3  Phase=pi/2  SampleTime=0
  x : Outport
  y : Outport  Port=2
  z : Outport  Port=3
  wires:
  Sine Wave y1 cercle/1 -> Product1/1
  Sine Wave x2 cercle/1 -> Product/2
  Sine Wave x1 cercle/1 -> Product/1
  Sine Wave y2 cercle/1 -> Product1/2
  Product/1 -> x/1
  Product1/1 -> y/1
  Sine Wave z1 cercle/1 -> z/1
